simulink model "Unbatch2_Model"  (R2024b)
settings: Solver=VariableStepAuto  StartTime=0.0  StopTime=10.0  RelTol=1e-3
libraries: NSA_DEVS_LOGISTICS x7, NSA_DEVS_SINKS x5, NSA_DEVS_SOURCES x2, NSA_DEVS_ROUTING x1
settings Model: Creator=david  LastModifiedBy=peter
settings RTWCC: GPUComputeCapability=3.5

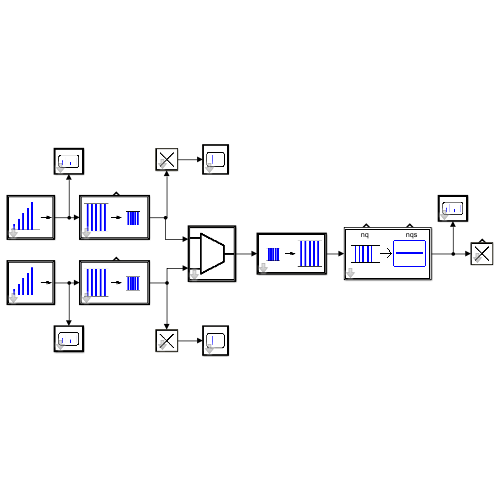
[thumbnail: Simulink's stored preview of the top-level diagram]
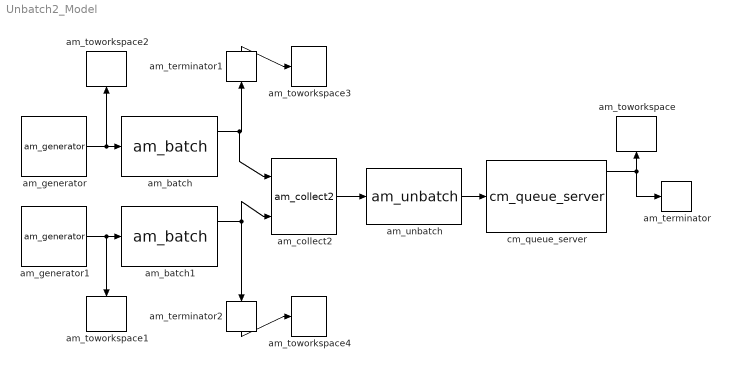
== system Unbatch2_Model ==
  am_batch : NSA_DEVS_LOGISTICS/am_batch  N=2  tau=[0,1]  debug=0
      settings: SourceProductName=Logistics
  am_batch1 : NSA_DEVS_LOGISTICS/am_batch  N=4  tau=[0,1]  debug=0
      settings: SourceProductName=Logistics
  am_collect2 : NSA_DEVS_ROUTING/am_collect2  tD=[0,2]  tau=[0,1]  debug=0
      settings: SourceProductName=Routing
  am_generator : NSA_DEVS_SOURCES/am_generator  tG=1  n0=0  nG=10  tD=[0,2]  debug=0
      settings: SourceProductName=Sources
  am_generator1 : NSA_DEVS_SOURCES/am_generator  tG=1  n0=10  nG=10  tD=[0,2]  debug=0
      settings: SourceProductName=Sources
  am_terminator : NSA_DEVS_LOGISTICS/am_terminator  tau=[0,1]  debug=0
      settings: SourceProductName=Logistics
  am_terminator1 : NSA_DEVS_LOGISTICS/am_terminator  tau=[0,1]  debug=0
      settings: SourceProductName=Logistics
  am_terminator2 : NSA_DEVS_LOGISTICS/am_terminator  tau=[0,1]  debug=0
      settings: SourceProductName=Logistics
  am_toworkspace : NSA_DEVS_SINKS/am_toworkspace  varname="\"out\""  t0=0  format="\"vector\""  tau=[0,0.5]  debug=0
      settings: SourceProductName=Sinks
  am_toworkspace1 : NSA_DEVS_SINKS/am_toworkspace  varname="\"in2\""  t0=0  format="\"vector\""  tau=[0,0.5]  debug=0
      settings: SourceProductName=Sinks
  am_toworkspace2 : NSA_DEVS_SINKS/am_toworkspace  varname="\"in1\""  t0=0  format="\"vector\""  tau=[0,0.5]  debug=0
      settings: SourceProductName=Sinks
  am_toworkspace3 : NSA_DEVS_SINKS/am_toworkspace  varname="\"batch1\""  t0=0  format="\"vector\""  tau=[0,0.5]  debug=0
      settings: SourceProductName=Sinks
  am_toworkspace4 : NSA_DEVS_SINKS/am_toworkspace  varname="\"batch2\""  t0=0  format="\"vector\""  tau=[0,0.5]  debug=0
      settings: SourceProductName=Sinks
  am_unbatch : NSA_DEVS_LOGISTICS/am_unbatch  tD=[0,2]  tau=[0,1]  debug=0
      settings: SourceProductName=Logistics
  cm_queue_server : NSA_DEVS_LOGISTICS/cm_queue_server  ts=0.1  tau=[0,1]  debug=0
      settings: SourceProductName=Logistics
  wires:
  am_generator/1 -> am_batch/1, am_toworkspace2/1
  am_generator1/1 -> am_toworkspace1/1, am_batch1/1
  am_collect2/1 -> am_unbatch/1
  am_terminator1/1 -> am_toworkspace3/1
  am_terminator2/1 -> am_toworkspace4/1
  am_unbatch/1 -> cm_queue_server/1
  cm_queue_server/1 -> am_toworkspace/1, am_terminator/1
  am_batch/1 -> am_collect2/1, am_terminator1/1
  am_batch1/1 -> am_collect2/2, am_terminator2/1
